simulink model "TF"  (R2021a)
settings: Solver=VariableStepAuto  StartTime=0.0  StopTime=inf  RelTol=1e-3
undefined symbols (not defined in the file or in its folder): MAV
settings Model: Creator=DELL  LastModifiedBy=DELL

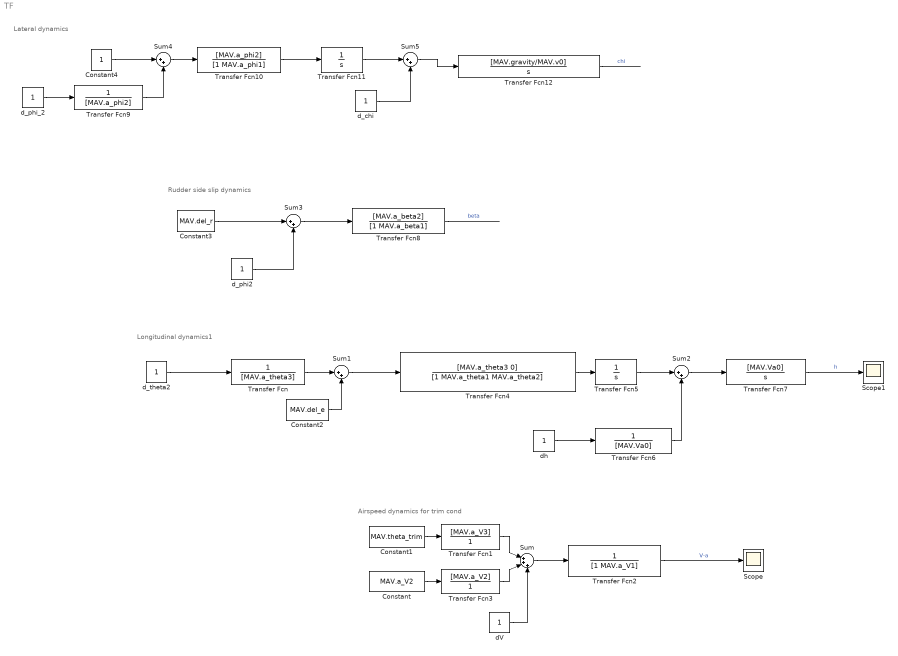
== system TF ==
  note: Lateral dynamics
  note: Rudder side slip dynamics
  note: Longitudinal dynamics1
  note: Airspeed dynamics for trim cond
  Constant : Constant  Value=MAV.a_V2
  Constant1 : Constant  Value=MAV.theta_trim
  Constant2 : Constant  Value=MAV.del_e
  Constant3 : Constant  Value=MAV.del_r
  Constant4 : Constant
  Scope : Scope
  Scope1 : Scope
  Sum : Sum  Inputs=|+++
  Sum{1..5} (5 alike) : Sum  Inputs=|++
  Transfer Fcn : TransferFcn  Denominator=[MAV.a_theta3]
  Transfer Fcn1 : TransferFcn  Numerator=[MAV.a_V3]  Denominator=[1]
  Transfer Fcn10 : TransferFcn  Numerator=[MAV.a_phi2]  Denominator=[1 MAV.a_phi1]
  Transfer Fcn11 : TransferFcn  Denominator=[1 0]
  Transfer Fcn12 : TransferFcn  Numerator=[MAV.gravity/MAV.v0]  Denominator=[1 0]
  Transfer Fcn2 : TransferFcn  Denominator=[1 MAV.a_V1]
  Transfer Fcn3 : TransferFcn  Numerator=[MAV.a_V2]  Denominator=[1]
  Transfer Fcn4 : TransferFcn  Numerator=[MAV.a_theta3 0]  Denominator=[1 MAV.a_theta1 MAV.a_theta2]
  Transfer Fcn5 : TransferFcn  Denominator=[1 0]
  Transfer Fcn6 : TransferFcn  Denominator=[MAV.Va0]
  Transfer Fcn7 : TransferFcn  Numerator=[MAV.Va0]  Denominator=[1 0]
  Transfer Fcn8 : TransferFcn  Numerator=[MAV.a_beta2]  Denominator=[1 MAV.a_beta1]
  Transfer Fcn9 : TransferFcn  Denominator=[MAV.a_phi2]
  dV : Constant
  d_chi : Constant
  d_phi2 : Constant
  d_phi_2 : Constant
  d_theta2 : Constant
  dh : Constant
  wires:
  Transfer Fcn2/1 -> Scope/1  "V-a"
  Transfer Fcn1/1 -> Sum/1
  Constant/1 -> Transfer Fcn3/1
  Transfer Fcn3/1 -> Sum/2
  dV/1 -> Sum/3
  Sum/1 -> Transfer Fcn2/1
  Constant1/1 -> Transfer Fcn1/1
  dh/1 -> Transfer Fcn6/1
  Sum2/1 -> Transfer Fcn7/1
  Transfer Fcn/1 -> Sum1/1
  Transfer Fcn4/1 -> Transfer Fcn5/1
  Constant2/1 -> Sum1/2
  d_theta2/1 -> Transfer Fcn/1
  Sum1/1 -> Transfer Fcn4/1
  Transfer Fcn6/1 -> Sum2/2
  Transfer Fcn5/1 -> Sum2/1
  Transfer Fcn7/1 -> Scope1/1  "h"
  Transfer Fcn8/1 -> ?  "beta"
  Constant3/1 -> Sum3/1
  Sum3/1 -> Transfer Fcn8/1
  d_phi2/1 -> Sum3/2
  Transfer Fcn12/1 -> ?  "chi"
  d_chi/1 -> Sum5/2
  Transfer Fcn11/1 -> Sum5/1
  Constant4/1 -> Sum4/1
  Sum5/1 -> Transfer Fcn12/1
  Transfer Fcn9/1 -> Sum4/2
  d_phi_2/1 -> Transfer Fcn9/1
  Sum4/1 -> Transfer Fcn10/1
  Transfer Fcn10/1 -> Transfer Fcn11/1
